simulink model "Lab4_simulink"  (R2024a)
settings: Solver=VariableStepAuto  StartTime=0.0  StopTime=10.0  MaxStep=0.1  RelTol=1e-3
values from neighbouring files (symbols this model uses):
  A = [0, 1 ... (first row only)    [Lab4.m]
  ALPHA = inv(-(C-D*K)*inv((A-B*K))*B+D)    [Lab4.m]
  B = [0 ... (first row only)    [Lab4.m]
  C = [Kt, 0]    [Lab4.m]
  D = 0    [Lab4.m]
  g = 9.81    [Lab4.m]
  Im = Im0    (= 0.8)    [Lab4.m]
  K = place(A,B,lambdaK)    [Lab4.m]
  Km = 1.52 * 10^(-4)    (= 0.000152)    [Lab4.m]
  Kt = 708.27    [Lab4.m]
  L = place(A',C',lambdaL)'    [Lab4.m]
  m = 0.02    [Lab4.m]
  x_ = 0.022    [Lab4.m]
settings Model: Creator=luigi  LastModifiedBy=luigi

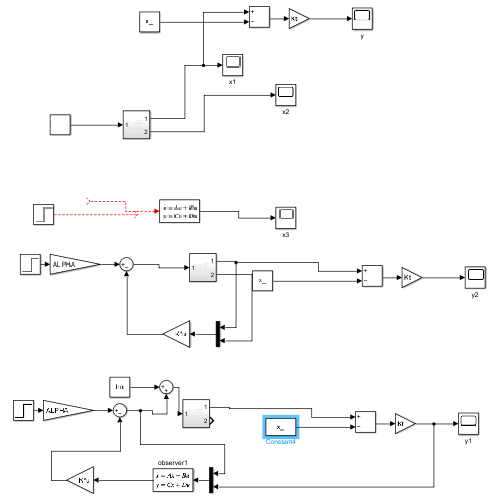
[thumbnail: Simulink's stored preview of the top-level diagram]
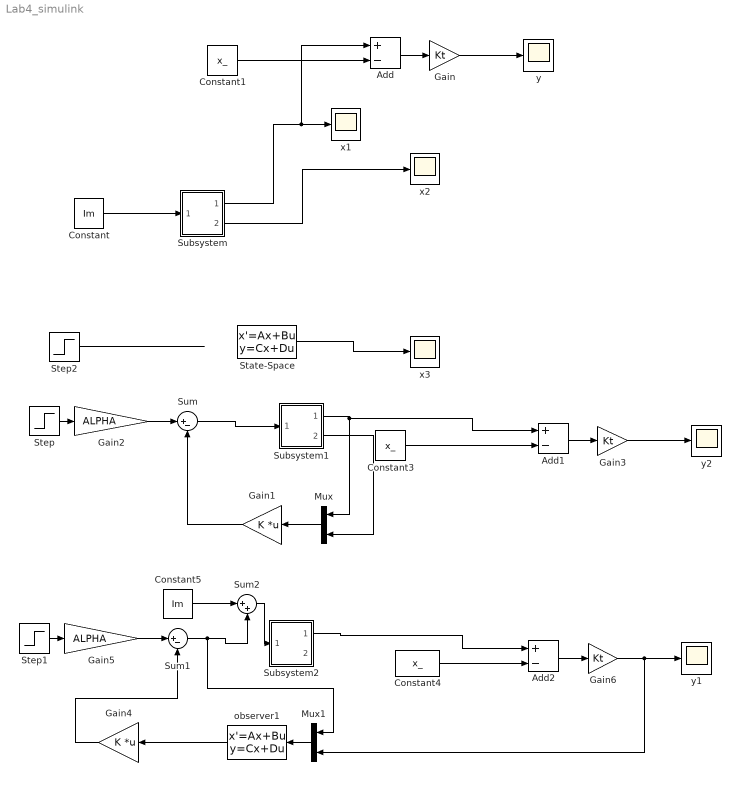
== system Lab4_simulink ==
  Add : Sum  Inputs=+-
  Add1 : Sum  Inputs=+-
  Add2 : Sum  Inputs=+-
  Constant : Constant  Value=Im
  Constant1 : Constant  Value=x_
  Constant3 : Constant  Value=x_
  Constant4 : Constant  Value=x_
  Constant5 : Constant  Value=Im
  Gain : Gain  Gain=Kt
  Gain1 : Gain  Gain=K  Multiplication=Matrix(K*u)
  Gain2 : Gain  Gain=ALPHA
  Gain3 : Gain  Gain=Kt
  Gain4 : Gain  Gain=K  Multiplication=Matrix(K*u)
  Gain5 : Gain  Gain=ALPHA
  Gain6 : Gain  Gain=Kt
  Mux : Mux  Inputs=2
  Mux1 : Mux  Inputs=2
  State-Space : StateSpace  A=[A-B*K, -B*K;zeros(2,2), A-L*C]  B=[B;zeros(2,1)]*ALPHA  C=[C-D*K, -D*K]  D=zeros(1,1)  InitialCondition=0
  Step : Step  Time=0  SampleTime=0
  Step1 : Step  Time=0  SampleTime=0
  Step2 : Step  Time=0  SampleTime=0
  Subsystem : Subsystem
  Subsystem1 : Subsystem
  Subsystem2 : Subsystem
  Sum : Sum  Inputs=|+-
  Sum1 : Sum  Inputs=|+-
  Sum2 : Sum  Inputs=|++
  observer1 : StateSpace  A=A-L*C  B="[B  L]"  C=eye(2)  D=zeros(2,2)  InitialCondition=[0 0]'
  x1 : Scope
  x2 : Scope
  x3 : Scope
  y : Scope
  y1 : Scope
  y2 : Scope
  wires:
  Constant/1 -> Subsystem/1(In1)
  Subsystem/1(Out1) -> x1/1, Add/1
  Subsystem/2(Out2) -> x2/1
  Constant1/1 -> Add/2
  Add/1 -> Gain/1
  Gain/1 -> y/1
  ? -> State-Space/1
  State-Space/1 -> x3/1
  Mux/1 -> Gain1/1
  Gain1/1 -> Sum/2
  Step/1 -> Gain2/1
  Gain2/1 -> Sum/1
  Sum/1 -> Subsystem1/1(In1)
  Subsystem1/1(Out2) -> Add1/1, Mux/1
  Subsystem1/2(Out1) -> Mux/2
  Gain3/1 -> y2/1
  Add1/1 -> Gain3/1
  Constant3/1 -> Add1/2
  Subsystem2/1(Out2) -> Add2/1
  Constant4/1 -> Add2/2
  Add2/1 -> Gain6/1
  Gain6/1 -> Mux1/2, y1/1
  Sum1/1 -> Mux1/1, Sum2/2
  Step1/1 -> Gain5/1
  Gain4/1 -> Sum1/2
  Gain5/1 -> Sum1/1
  Mux1/1 -> observer1/1
  observer1/1 -> Gain4/1
  Sum2/1 -> Subsystem2/1(In1)
  Constant5/1 -> Sum2/1
  Step2/1 -> ?

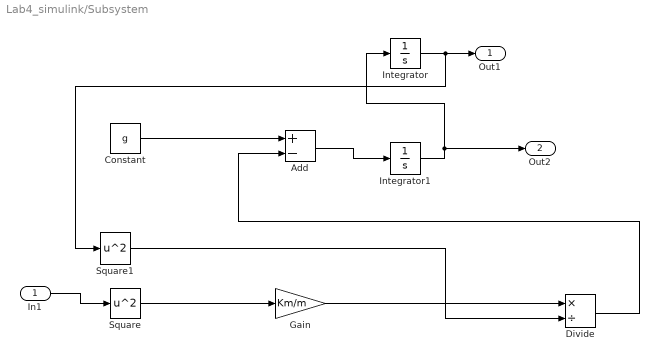
== system Lab4_simulink/Subsystem ==
  In1 : Inport
  Add : Sum  Inputs=+-
  Constant : Constant  Value=g
  Divide : Product  Inputs=*/
  Gain : Gain  Gain=Km/m
  Integrator : Integrator  InitialCondition=x_+0.01
  Integrator1 : Integrator
  Square : Math  Operator=square
  Square1 : Math  Operator=square
  Out1 : Outport
  Out2 : Outport  Port=2
  wires:
  Integrator/1 -> Out1/1, Square1/1
  Square/1 -> Gain/1
  Add/1 -> Integrator1/1
  Square1/1 -> Divide/2
  Integrator1/1 -> Out2/1, Integrator/1
  In1/1 -> Square/1
  Divide/1 -> Add/2
  Constant/1 -> Add/1
  Gain/1 -> Divide/1

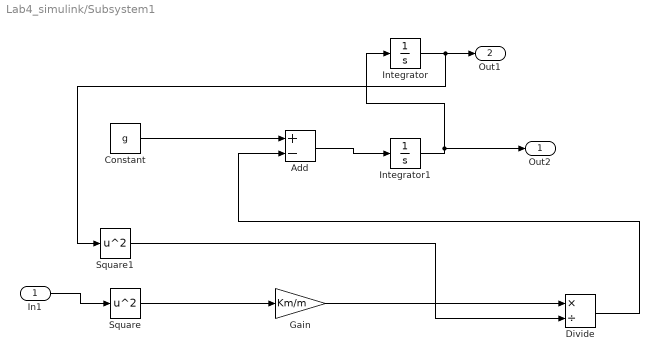
== system Lab4_simulink/Subsystem1 ==
  In1 : Inport
  Add : Sum  Inputs=+-
  Constant : Constant  Value=g
  Divide : Product  Inputs=*/
  Gain : Gain  Gain=Km/m
  Integrator : Integrator  InitialCondition=x_+0.01
  Integrator1 : Integrator
  Square : Math  Operator=square
  Square1 : Math  Operator=square
  Out2 : Outport
  Out1 : Outport  Port=2
  wires:
  Integrator/1 -> Out1/1, Square1/1
  Square/1 -> Gain/1
  Add/1 -> Integrator1/1
  Square1/1 -> Divide/2
  Integrator1/1 -> Out2/1, Integrator/1
  In1/1 -> Square/1
  Divide/1 -> Add/2
  Constant/1 -> Add/1
  Gain/1 -> Divide/1

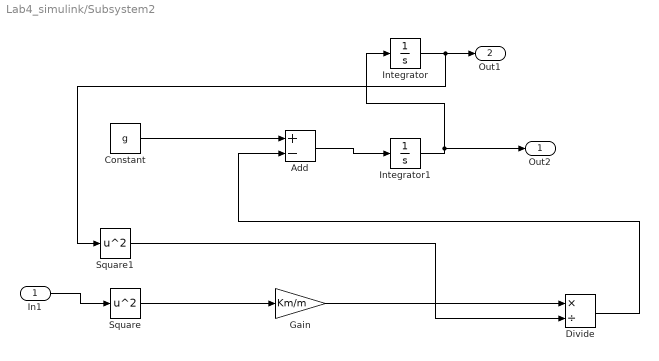
== system Lab4_simulink/Subsystem2 ==
  In1 : Inport
  Add : Sum  Inputs=+-
  Constant : Constant  Value=g
  Divide : Product  Inputs=*/
  Gain : Gain  Gain=Km/m
  Integrator : Integrator  InitialCondition=x_
  Integrator1 : Integrator
  Square : Math  Operator=square
  Square1 : Math  Operator=square
  Out2 : Outport
  Out1 : Outport  Port=2
  wires:
  Integrator/1 -> Out1/1, Square1/1
  Square/1 -> Gain/1
  Add/1 -> Integrator1/1
  Square1/1 -> Divide/2
  Integrator1/1 -> Out2/1, Integrator/1
  In1/1 -> Square/1
  Divide/1 -> Add/2
  Constant/1 -> Add/1
  Gain/1 -> Divide/1
